simulink model "TEMs_CAR"  (R2015a)
settings: Solver=ode3  StartTime=0.0  StopTime=1372  FixedStep=1  RelTol=5e-3
values from neighbouring files (symbols this model uses):
  a = 0.062*0.062    (= 0.003844)    [TEM_CAR.m]
  a_hxr = 0.0127    [TEM_CAR.m]
  B = 0.45*0.16/5    (= 0.0144)    [TEM_CAR.m]
  b_hxr = 0.16    [TEM_CAR.m]
  C_ap = 900    [TEM_CAR.m]
  C_cxr = 950    [TEM_CAR.m]
  C_hxr = 500    [TEM_CAR.m]
  ca1 = 0.99971*9*1.2    (= 10.796868)    [TEM_CAR.m]
  ca2 = 0.00021632    [TEM_CAR.m]
  ca3 = 0.33723    [TEM_CAR.m]
  cb1 = 0.023    [TEM_CAR.m]
  cb2 = 0.8    [TEM_CAR.m]
  cb3 = 0.33    [TEM_CAR.m]
  ct1 = 6.3195*1.2    (= 7.5834)    [TEM_CAR.m]
  ct2 = -5.337*1.2    (= -6.4044)    [TEM_CAR.m]
  Di_cxr = 2*0.0889*(0.01-2*0.0015)/(0.0889+0.01-2*0.0015)    (= 0.0129781021898)    [TEM_CAR.m]
  f = 2*127*0.0028*0.0028/(0.062*0.062)    (= 0.518043704475)    [TEM_CAR.m]
  l = 1e-3    (= 0.001)    [TEM_CAR.m]
  l_cw = 1.5e-3    (= 0.0015)    [TEM_CAR.m]
  l_hxr = 0.45/6    (= 0.075)    [TEM_CAR.m]
  M = 2    [TEM_CAR.m]
  M_ap = 0.024066*3    (= 0.072198)    [TEM_CAR.m]
  m_col = 0.2    [TEM_CAR.m]
  M_cxr = 1.5045*3    (= 4.5135)    [TEM_CAR.m]
  M_hxr = 0.16128*3    (= 0.48384)    [TEM_CAR.m]
  n = 127    [TEM_CAR.m]
  Nf_hxr = 13*4.5    (= 58.5)    [TEM_CAR.m]
  r_int = 6-0.4    (= 5.6)    [TEM_CAR.m]
  side = 2    [TEM_CAR.m]
  T_cint = 286    [TEM_CAR.m]
  T_hint = 306.64    [TEM_CAR.m]
  tf_hxr = 0.00032    [TEM_CAR.m]
  Tune_er = 0.5    [TEM_CAR.m]
  Tune_tr = 1    [TEM_CAR.m]
undefined symbols (not defined in the file or in its folder): k_gap, N, P, plate_fin_hxr_A, T1, T1_T2
libraries: LU_TEG x8
(part 2 of 2)

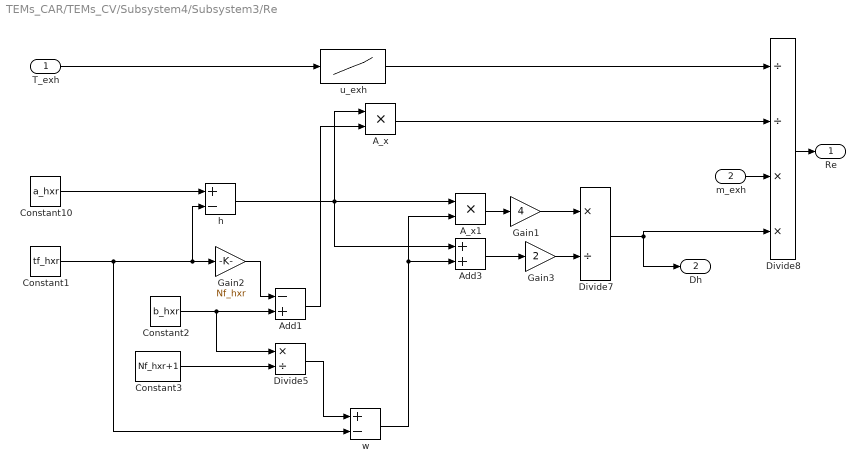
== system TEMs_CAR/TEMs_CV/Subsystem4/Subsystem3/Re ==
  T_exh : Inport
  m_exh : Inport  Port=2
  A_x : Product  Inputs=**
  A_x1 : Product  Inputs=**
  Add1 : Sum  Inputs=-+
  Add3 : Sum
  Constant1 : Constant  Value=tf_hxr
  Constant10 : Constant  Value=a_hxr
  Constant2 : Constant  Value=b_hxr
  Constant3 : Constant  Value=Nf_hxr+1
  Divide5 : Product  Inputs=*/
  Divide7 : Product  Inputs=*/
  Divide8 : Product  Inputs=//**
  Gain1 : Gain  Gain=4
  Gain2 : Gain  Gain=Nf_hxr
  Gain3 : Gain  Gain=2
  h : Sum  Inputs=+-
  u_exh : Lookup_n-D  NumberOfTableDimensions=1  BreakpointsForDimension1=|  Table=|  InterpMethod=Cubic spline  ExtrapMethod=Cubic spline  RndMeth=Simplest  InputSameDT=on
      BreakpointsForDimension1=|
      | [293
      | 313
      | 333
      | 353
      | 373
      | 393
      | 413
      | 433
      | 453
      | 473
      | 493
      | 513
      | 533
      | 553
      | 573
      | 593
      | 613
      | 633
      | 653
      | 673
      | 693
      | 713
      | 733
      | 753
      | 773
      | 793
      | 813
      | 833
      | 853
      | 873
      | 900
      | 920
      | 940
      | 960
      | 980
      | 1000
      | 1020
      | 1040
      | 1060
      | 1080
      | 1100
      | 1120
      | 1140
      | 1160
      | 1180
      | 1200
      | 1220
      | 1240
      | 1260
      | 1280
      | 1300
      | 1320
      | 1340
      | 1360
      | 1380
      | 1400
      | 1420
      | 1440
      | 1460
      | 1480
      | ]
      Table=|
      | [1.81E-05
      | 1.91E-05
      | 2.00E-05
      | 2.09E-05
      | 2.17E-05
      | 2.26E-05
      | 2.34E-05
      | 2.42E-05
      | 2.50E-05
      | 2.57E-05
      | 2.64E-05
      | 2.72E-05
      | 2.79E-05
      | 2.86E-05
      | 2.93E-05
      | 2.99E-05
      | 3.06E-05
      | 3.12E-05
      | 3.19E-05
      | 3.25E-05
      | 3.31E-05
      | 3.37E-05
      | 3.43E-05
      | 3.49E-05
      | 3.55E-05
      | 3.60E-05
      | 3.66E-05
      | 3.72E-05
      | 3.77E-05
      | 3.82E-05
      | 3.90E-05
      | 3.95E-05
      | 4.00E-05
      | 4.05E-05
      | 4.10E-05
      | 4.15E-05
      | 4.20E-05
      | 4.25E-05
      | 4.30E-05
      | 4.35E-05
      | 4.40E-05
      | 4.44E-05
      | 4.49E-05
      | 4.53E-05
      | 4.58E-05
      | 4.63E-05
      | 4.67E-05
      | 4.71E-05
      | 4.76E-05
      | 4.80E-05
      | 4.85E-05
      | 4.89E-05
      | 4.93E-05
      | 4.97E-05
      | 5.02E-05
      | 5.06E-05
      | 5.10E-05
      | 5.14E-05
      | 5.18E-05
      | 5.22E-05
      | ]
  w : Sum  Inputs=+-
  Re : Outport
  Dh : Outport  Port=2
  wires:
  Divide8/1 -> Re/1
  T_exh/1 -> u_exh/1
  Constant10/1 -> h/1
  h/1 -> Add3/1, A_x1/1, A_x/1
  Constant2/1 -> Divide5/1, Add1/2
  Gain2/1 -> Add1/1
  Add1/1 -> A_x/2
  Constant3/1 -> Divide5/2
  Divide5/1 -> w/1
  Constant1/1 -> w/2, h/2, Gain2/1
  w/1 -> A_x1/2, Add3/2
  Gain1/1 -> Divide7/1
  Gain3/1 -> Divide7/2
  Add3/1 -> Gain3/1
  Divide7/1 -> Divide8/4, Dh/1
  u_exh/1 -> Divide8/1
  A_x/1 -> Divide8/2
  m_exh/1 -> Divide8/3
  A_x1/1 -> Gain1/1

== system TEMs_CAR/TEMs_CV/Subsystem5/Subsystem3/Re ==
  T_col : Inport
  m_col : Inport  Port=2
  Constant : Constant  Value=4/pi/Di_cxr
  Divide8 : Product  Inputs=/**
  u_col : Lookup_n-D  NumberOfTableDimensions=1  BreakpointsForDimension1=|  Table=|  InterpMethod=Cubic spline  ExtrapMethod=Cubic spline  RndMeth=Simplest  InputSameDT=on
      BreakpointsForDimension1=|
      | [273
      | 274
      | 275
      | 276
      | 277
      | 278
      | 279
      | 280
      | 281
      | 282
      | 283
      | 284
      | 285
      | 286
      | 287
      | 288
      | 289
      | 290
      | 291
      | 292
      | 293
      | 294
      | 295
      | 296
      | 297
      | 298
      | 299
      | 300
      | 301
      | 302
      | 303
      | 304
      | 305
      | 306
      | 307
      | 308
      | 309
      | 310
      | 311
      | 312
      | 313
      | 314
      | 315
      | 316
      | 317
      | 318
      | 319
      | 320
      | 321
      | 322
      | 323
      | 324
      | 325
      | 326
      | 327
      | 328
      | 329
      | 330
      | 331
      | 332
      | 333
      | 334
      | 335
      | 336
      | 337
      | 338
      | 339
      | 340
      | 341
      | 342
      | 343
      | 344
      | 345
      | 346
      | 347
      | 348
      | 349
      | 350
      | 351
      | 352
      | 353
      | 354
      | 355
      | 356
      | 357
      | 358
      | 359
      | 360
      | 361
      | 362
      | 363
      | 364
      | 365
      | 366
      | 367
      | 368
      | 369
      | 370
      | 371
      | 372
      | 373]
      Table=|
      | [0.001792
      | 0.001731
      | 0.001674
      | 0.00162
      | 0.001569
      | 0.00152
      | 0.001473
      | 0.001429
      | 0.001386
      | 0.001346
      | 0.001308
      | 0.001271
      | 0.001236
      | 0.001202
      | 0.00117
      | 0.001139
      | 0.001109
      | 0.001081
      | 0.001054
      | 0.001028
      | 0.001003
      | 0.000979
      | 0.000955
      | 0.000933
      | 0.000911
      | 0.000891
      | 0.000871
      | 0.000852
      | 0.000833
      | 0.000815
      | 0.000798
      | 0.000781
      | 0.000765
      | 0.000749
      | 0.000734
      | 0.00072
      | 0.000705
      | 0.000692
      | 0.000678
      | 0.000666
      | 0.000653
      | 0.000641
      | 0.000629
      | 0.000618
      | 0.000607
      | 0.000596
      | 0.000586
      | 0.000576
      | 0.000566
      | 0.000556
      | 0.000547
      | 0.000538
      | 0.000529
      | 0.000521
      | 0.000512
      | 0.000504
      | 0.000496
      | 0.000489
      | 0.000481
      | 0.000474
      | 0.000467
      | 0.00046
      | 0.000453
      | 0.000447
      | 0.00044
      | 0.000434
      | 0.000428
      | 0.000422
      | 0.000416
      | 0.00041
      | 0.000404
      | 0.000399
      | 0.000394
      | 0.000388
      | 0.000383
      | 0.000378
      | 0.000373
      | 0.000369
      | 0.000364
      | 0.000359
      | 0.000355
      | 0.000351
      | 0.000346
      | 0.000342
      | 0.000338
      | 0.000334
      | 0.00033
      | 0.000326
      | 0.000322
      | 0.000319
      | 0.000315
      | 0.000311
      | 0.000308
      | 0.000304
      | 0.000301
      | 0.000298
      | 0.000295
      | 0.000291
      | 0.000288
      | 0.000285
      | 0.000282
      | ]
  Re : Outport
  wires:
  Constant/1 -> Divide8/3
  m_col/1 -> Divide8/2
  Divide8/1 -> Re/1
  T_col/1 -> u_col/1
  u_col/1 -> Divide8/1
